simulink model "ApplicationSwComponentType11"  (R2024b)
settings: Solver=FixedStepDiscrete  StartTime=0.0  StopTime=10.0  FixedStep=0.01  RelTol=1e-3
model workspace (MAT data in the model file):
  ArTypedPerInstanceMemory = Simulink.Signal
  ArTypedPerInstanceMemory.Dimensions = 1
  ArTypedPerInstanceMemory.DimensionsMode = 'auto'
  ArTypedPerInstanceMemory.Complexity = 'real'
  ArTypedPerInstanceMemory.SampleTime = -1
  ArTypedPerInstanceMemory.SamplingMode = 'auto'
  ArTypedPerInstanceMemory.InitialValue = '-3'
  ArTypedPerInstanceMemory.DataType = 'int16'
  ConstantMemory = Simulink.Parameter
  ConstantMemory.Value = 3
  ConstantMemory.Complexity = 'real'
  ConstantMemory.Dimensions = [1 1]
  ConstantMemory.DataType = 'uint64'
  PerInstanceParameter = Simulink.Parameter
  PerInstanceParameter.Value = 5
  PerInstanceParameter.Complexity = 'real'
  PerInstanceParameter.Dimensions = [1 1]
  PerInstanceParameter.DataType = 'uint8'
  RPort_prm_Parameter = Simulink.Parameter
  RPort_prm_Parameter.Value = 0
  RPort_prm_Parameter.Complexity = 'real'
  RPort_prm_Parameter.Dimensions = [1 1]
  RPort_prm_Parameter.DataType = 'single'
  RPort_prm_Parameter1 = Simulink.Parameter
  RPort_prm_Parameter1.Value = 0
  RPort_prm_Parameter1.Complexity = 'real'
  RPort_prm_Parameter1.Dimensions = [1 1]
  RPort_prm_Parameter1.DataType = 'uint8'
  SharedParameter = Simulink.Parameter
  SharedParameter.Value = 5.5
  SharedParameter.Complexity = 'real'
  SharedParameter.Dimensions = [1 1]
  SharedParameter.DataType = 'single'
  StaticMemory = Simulink.Signal
  StaticMemory.Dimensions = 1
  StaticMemory.DimensionsMode = 'auto'
  StaticMemory.Complexity = 'real'
  StaticMemory.SampleTime = -1
  StaticMemory.SamplingMode = 'auto'
  StaticMemory.InitialValue = '9'
  StaticMemory.DataType = 'uint8'
settings Model: ParameterArgumentNames=PerInstanceParameter,RPort_prm_Parameter,RPort_prm_Parameter1  Creator=sss923875  LastModifiedBy=sss923875
settings DataIOCC: SaveFormat=StructureWithTime
settings OptimizationCC: DefaultParameterBehavior=Inlined  EnhancedBackFolding=on  PassReuseOutputArgsAs=Individual arguments  ZeroExternalMemoryAtStartup=off  ZeroInternalMemoryAtStartup=off  OptimizeBlockOrder=speed  DifferentSizesBufferReuse=on  OptimizationCustomize=off  EfficientTunableParamExpr=on
settings DebuggingCC: ParameterTunabilityLossMsg=error
settings HardwareCC: ProdLongLongMode=on
settings ModelReferenceCC: ModelReferenceNumInstancesAllowed=Single
settings SFSimCC: MATLABDynamicMemAlloc=off
settings RTWCC: Description=AUTOSAR  SystemTargetFile=autosar.tlc  GenCodeOnly=on  TemplateMakefile=ert_default_tmf  DataTypeReplacement=CDataTypesFixedWidth
settings CodeAppCC: ForceParamTrailComments=on  IgnoreCustomStorageClasses=off  OperatorAnnotations=on  SimulinkDataObjDesc=on  SFDataObjDesc=on  InsertBlockDesc=on
settings STFCustomTargetCC: TargetLangStandard=C99 (ISO)  MultiwordLength=256  ParMdlRefBuildCompliant=on  CompOptLevelCompliant=on  IncludeMdlTerminateFcn=off  CombineOutputUpdateFcns=on  SuppressErrorStatus=on  ERTCustomFileBanners=on  SupportNonFinite=off  SupportComplex=off  SupportContinuousTime=off  SupportNonInlinedSFcns=off  RemoveResetFunc=on  MATLABClassNameForMDSCustomization=Simulink.SoftwareTarget.ERTCustomization  AutosarCompliant=on  UseToolchainInfoCompliant=on  LookupTableObjectStructAxisOrder=2,1,3,4,...  LUTObjectStructOrderEvenSpacing=Size,Table,Breakpoints  SystemTargetFile=autosar.tlc
settings ERTTargetCC: TargetLangStandard=C99 (ISO)  ConcurrentExecutionCompliant=off  IncludeMdlTerminateFcn=off  SuppressErrorStatus=on  SupportNonFinite=off  SupportComplex=off  ModelStepFunctionPrototypeControlCompliant=off  CPPClassGenCompliant=off  AutosarCompliant=on  LookupTableObjectStructAxisOrder=2,1,3,4,...  LUTObjectStructOrderEvenSpacing=Size,Table,Breakpoints  ERTCustomFileTemplate=example_file_process.tlc  BooleanTrueId=TRUE  BooleanFalseId=FALSE

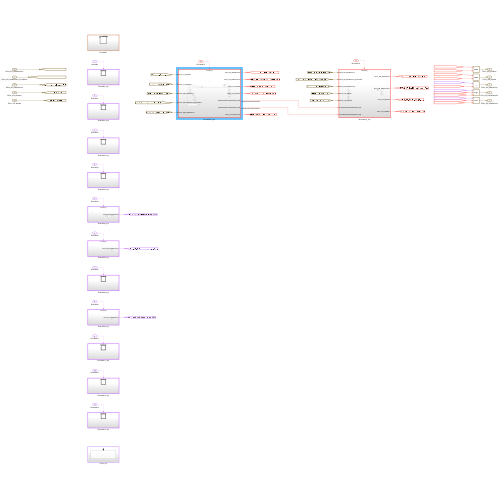
[thumbnail: Simulink's stored preview of the top-level diagram]
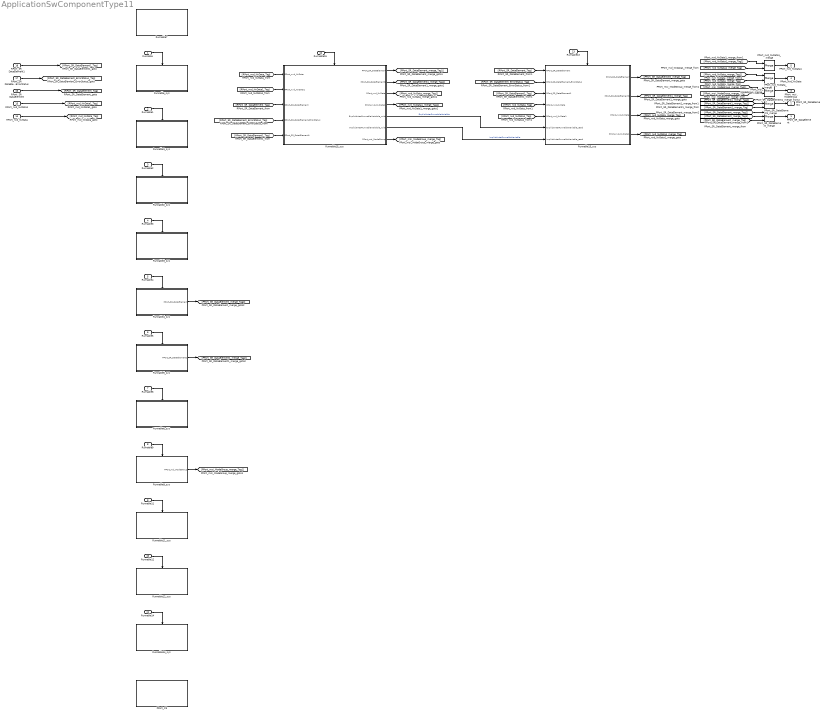
== system ApplicationSwComponentType11 ==
  Runnable : Inport  OutputFunctionCall=on
  Runnable1 : Inport  Port=2  OutputFunctionCall=on
  Runnable2 : Inport  Port=3  OutputFunctionCall=on
  Runnable3 : Inport  Port=4  OutputFunctionCall=on
  Runnable4 : Inport  Port=5  OutputFunctionCall=on
  Runnable5 : Inport  Port=6  OutputFunctionCall=on
  Runnable6 : Inport  Port=7  OutputFunctionCall=on
  Runnable9 : Inport  Port=8  OutputFunctionCall=on
  Runnable11 : Inport  Port=9  OutputFunctionCall=on
  Runnable12 : Inport  Port=10  OutputFunctionCall=on
  Runnable14 : Inport  Port=11  OutputFunctionCall=on
  Runnable15 : Inport  Port=12  SampleTime=0.01  OutputFunctionCall=on
  Runnable13 : Inport  Port=13  SampleTime=0.01  OutputFunctionCall=on
  RPort_nvd_NvData : Inport  Port=14  OutDataTypeStr=uint8  PortDimensions=1
  RPort_nvd_NvData1 : Inport  Port=15  OutDataTypeStr=double  PortDimensions=1
  RPort_SR_DataElement : Inport  Port=16  OutMin=0  OutMax=7  OutDataTypeStr=ApplicationPrimitiveDataType  PortDimensions=1
  RPort_SR_DataElement_ErrorStatus : Inport  Port=17  OutDataTypeStr=uint8  PortDimensions=1
  RPort_SR_DataElement1 : Inport  Port=18  OutDataTypeStr=uint32  PortDimensions=1
  PPort_CS : Subsystem
  PPort_SR_DataElement1_merge : Merge  Inputs=2+ 1
  PPort_SR_DataElement_merge : Merge  Inputs=2+ 1
  PPort_msi_ModeGroup_merge : Merge
  PPort_nvd_NvData1_merge : Merge
  PPort_nvd_NvData_merge : Merge
  Runnable11_sys : Subsystem
  Runnable12_sys : Subsystem
  Runnable13_sys : Subsystem
  Runnable14_sys : Subsystem
  Runnable15_sys : Subsystem
  Runnable1_sys : Subsystem
  Runnable2_sys : Subsystem
  Runnable3_sys : Subsystem
  Runnable4_sys : Subsystem
  Runnable5_sys : Subsystem
  Runnable6_sys : Subsystem
  Runnable7 : Subsystem
  Runnable9_sys : Subsystem
  Runnable_sys : Subsystem
  PPort_SR_DataElement : Outport  OutMin=0  OutMax=7  OutDataTypeStr=ApplicationPrimitiveDataType  PortDimensions=1
  PPort_SR_DataElement1 : Outport  Port=2  OutDataTypeStr=uint32  PortDimensions=1
  PPort_msi_ModeGroup : Outport  Port=3  OutDataTypeStr=Enum: ModeDeclarationGroup  PortDimensions=1
  PPort_nvd_NvData : Outport  Port=4  OutDataTypeStr=uint8  PortDimensions=1
  PPort_nvd_NvData1 : Outport  Port=5  OutDataTypeStr=double  PortDimensions=1
  wires:
  PPort_SR_DataElement_merge/1 -> PPort_SR_DataElement/1
  PPort_SR_DataElement1_merge/1 -> PPort_SR_DataElement1/1
  PPort_msi_ModeGroup_merge/1 -> PPort_msi_ModeGroup/1
  PPort_nvd_NvData_merge/1 -> PPort_nvd_NvData/1
  PPort_nvd_NvData1_merge/1 -> PPort_nvd_NvData1/1
  Runnable15_sys/5(ExplicitInterRunnableVariable_write) -> Runnable13_sys/6(ExplicitInterRunnableVariable_read)  "ExplicitInterRunnableVariable"
  Runnable15_sys/6(ImplicitInterRunnableVariable_write) -> Runnable13_sys/7(ImplicitInterRunnableVariable_read)  "ImplicitInterRunnableVariable"
  Runnable13_sys/4(PPort_nvd_NvData1) -> [PPort_nvd_NvData1_merge_Tag]
  [PPort_nvd_NvData1_merge_Tag] -> PPort_nvd_NvData1_merge/2
  Runnable15_sys/4(PPort_nvd_NvData1) -> [PPort_nvd_NvData1_merge_Tag1]
  [PPort_nvd_NvData1_merge_Tag1] -> PPort_nvd_NvData1_merge/1
  Runnable13_sys/3(PPort_nvd_NvData) -> [PPort_nvd_NvData_merge_Tag]
  [PPort_nvd_NvData_merge_Tag] -> PPort_nvd_NvData_merge/2
  Runnable15_sys/3(PPort_nvd_NvData) -> [PPort_nvd_NvData_merge_Tag1]
  [PPort_nvd_NvData_merge_Tag1] -> PPort_nvd_NvData_merge/1
  Runnable13_sys/2(PPort_SR_DataElement1) -> [PPort_SR_DataElement1_merge_Tag]
  [PPort_SR_DataElement1_merge_Tag] -> PPort_SR_DataElement1_merge/3
  Runnable13_sys/1(PPort_SR_DataElement) -> [PPort_SR_DataElement_merge_Tag]
  [PPort_SR_DataElement_merge_Tag] -> PPort_SR_DataElement_merge/3
  Runnable15_sys/7(PPort_msi_ModeGroup) -> [PPort_msi_ModeGroup_merge_Tag]
  [PPort_msi_ModeGroup_merge_Tag] -> PPort_msi_ModeGroup_merge/2
  Runnable9_sys/1(PPort_msi_ModeGroup) -> [PPort_msi_ModeGroup_merge_Tag1]
  [PPort_msi_ModeGroup_merge_Tag1] -> PPort_msi_ModeGroup_merge/1
  Runnable15_sys/2(PPort_SR_DataElement1) -> [PPort_SR_DataElement1_merge_Tag1]
  [PPort_SR_DataElement1_merge_Tag1] -> PPort_SR_DataElement1_merge/2
  Runnable5_sys/1(PPort_SR_DataElement1) -> [PPort_SR_DataElement1_merge_Tag2]
  [PPort_SR_DataElement1_merge_Tag2] -> PPort_SR_DataElement1_merge/1
  Runnable15_sys/1(PPort_SR_DataElement) -> [PPort_SR_DataElement_merge_Tag1]
  [PPort_SR_DataElement_merge_Tag1] -> PPort_SR_DataElement_merge/2
  Runnable4_sys/1(PPort_SR_DataElement) -> [PPort_SR_DataElement_merge_Tag2]
  [PPort_SR_DataElement_merge_Tag2] -> PPort_SR_DataElement_merge/1
  RPort_SR_DataElement1/1 -> [RPort_SR_DataElement1_Tag]
  [RPort_SR_DataElement1_Tag] -> Runnable15_sys/5(RPort_SR_DataElement1)
  [RPort_SR_DataElement1_Tag] -> Runnable13_sys/3(RPort_SR_DataElement1)
  RPort_SR_DataElement_ErrorStatus/1 -> [RPort_SR_DataElement_ErrorStatus_Tag]
  [RPort_SR_DataElement_ErrorStatus_Tag] -> Runnable15_sys/4(RPort_SR_DataElement_ErrorStatus)
  [RPort_SR_DataElement_ErrorStatus_Tag] -> Runnable13_sys/2(RPort_SR_DataElement_ErrorStatus)
  RPort_SR_DataElement/1 -> [RPort_SR_DataElement_Tag]
  [RPort_SR_DataElement_Tag] -> Runnable15_sys/3(RPort_SR_DataElement)
  [RPort_SR_DataElement_Tag] -> Runnable13_sys/1(RPort_SR_DataElement)
  RPort_nvd_NvData1/1 -> [RPort_nvd_NvData1_Tag]
  [RPort_nvd_NvData1_Tag] -> Runnable15_sys/2(RPort_nvd_NvData1)
  [RPort_nvd_NvData1_Tag] -> Runnable13_sys/5(RPort_nvd_NvData1)
  RPort_nvd_NvData/1 -> [RPort_nvd_NvData_Tag]
  [RPort_nvd_NvData_Tag] -> Runnable15_sys/1(RPort_nvd_NvData)
  [RPort_nvd_NvData_Tag] -> Runnable13_sys/4(RPort_nvd_NvData)
  Runnable/1 -> Runnable_sys/Trigger
  Runnable1/1 -> Runnable1_sys/Trigger
  Runnable2/1 -> Runnable2_sys/Trigger
  Runnable3/1 -> Runnable3_sys/Trigger
  Runnable4/1 -> Runnable4_sys/Trigger
  Runnable5/1 -> Runnable5_sys/Trigger
  Runnable6/1 -> Runnable6_sys/Trigger
  Runnable9/1 -> Runnable9_sys/Trigger
  Runnable11/1 -> Runnable11_sys/Trigger
  Runnable12/1 -> Runnable12_sys/Trigger
  Runnable14/1 -> Runnable14_sys/Trigger
  Runnable15/1 -> Runnable15_sys/Trigger
  Runnable13/1 -> Runnable13_sys/Trigger

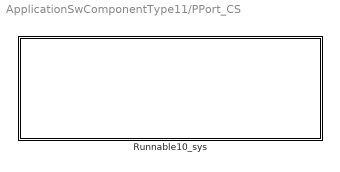
== system ApplicationSwComponentType11/PPort_CS ==
  Runnable10_sys : Subsystem

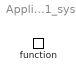
== system ApplicationSwComponentType11/Runnable11_sys ==
  function : TriggerPort  TriggerType=function-call  VariantControl=(inherit)

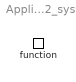
== system ApplicationSwComponentType11/Runnable12_sys ==
  function : TriggerPort  TriggerType=function-call  VariantControl=(inherit)

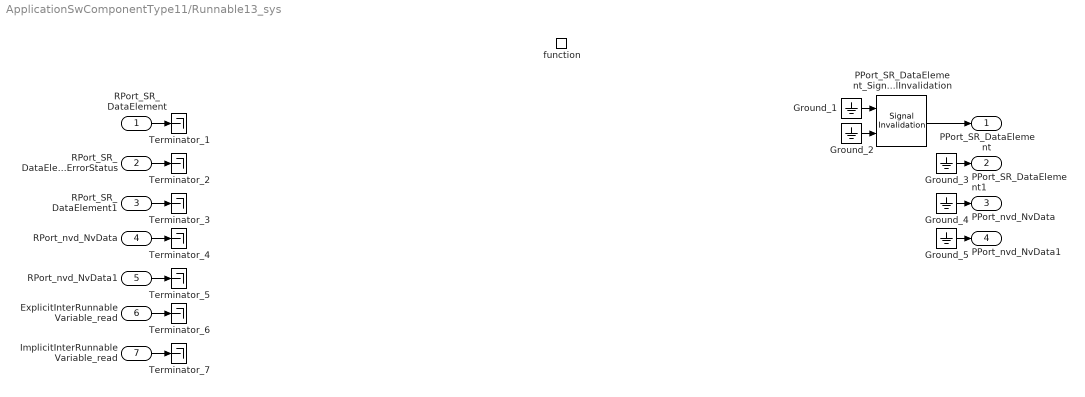
== system ApplicationSwComponentType11/Runnable13_sys ==
  RPort_SR_DataElement : Inport
  RPort_SR_DataElement_ErrorStatus : Inport  Port=2
  RPort_SR_DataElement1 : Inport  Port=3
  RPort_nvd_NvData : Inport  Port=4
  RPort_nvd_NvData1 : Inport  Port=5
  ExplicitInterRunnableVariable_read : Inport  Port=6
  ImplicitInterRunnableVariable_read : Inport  Port=7
  function : TriggerPort  TriggerType=function-call  VariantControl=(inherit)  SampleTimeType=periodic  SampleTime=-1
  Ground_{1..5} (5 alike) : Ground
  PPort_SR_DataElement_SignalInvalidation : SignalInvalidation
  Terminator_{1..7} (7 alike) : Terminator
  PPort_SR_DataElement : Outport
      settings: EnsureOutportIsVirtual=on
  PPort_SR_DataElement1 : Outport  Port=2
      settings: EnsureOutportIsVirtual=on
  PPort_nvd_NvData : Outport  Port=3
      settings: EnsureOutportIsVirtual=on
  PPort_nvd_NvData1 : Outport  Port=4
      settings: EnsureOutportIsVirtual=on
  wires:
  PPort_SR_DataElement_SignalInvalidation/1 -> PPort_SR_DataElement/1
  RPort_SR_DataElement/1 -> Terminator_1/1
  RPort_SR_DataElement_ErrorStatus/1 -> Terminator_2/1
  RPort_SR_DataElement1/1 -> Terminator_3/1
  RPort_nvd_NvData/1 -> Terminator_4/1
  RPort_nvd_NvData1/1 -> Terminator_5/1
  ExplicitInterRunnableVariable_read/1 -> Terminator_6/1
  ImplicitInterRunnableVariable_read/1 -> Terminator_7/1
  Ground_1/1 -> PPort_SR_DataElement_SignalInvalidation/1
  Ground_2/1 -> PPort_SR_DataElement_SignalInvalidation/2
  Ground_3/1 -> PPort_SR_DataElement1/1
  Ground_4/1 -> PPort_nvd_NvData/1
  Ground_5/1 -> PPort_nvd_NvData1/1

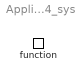
== system ApplicationSwComponentType11/Runnable14_sys ==
  function : TriggerPort  TriggerType=function-call  VariantControl=(inherit)

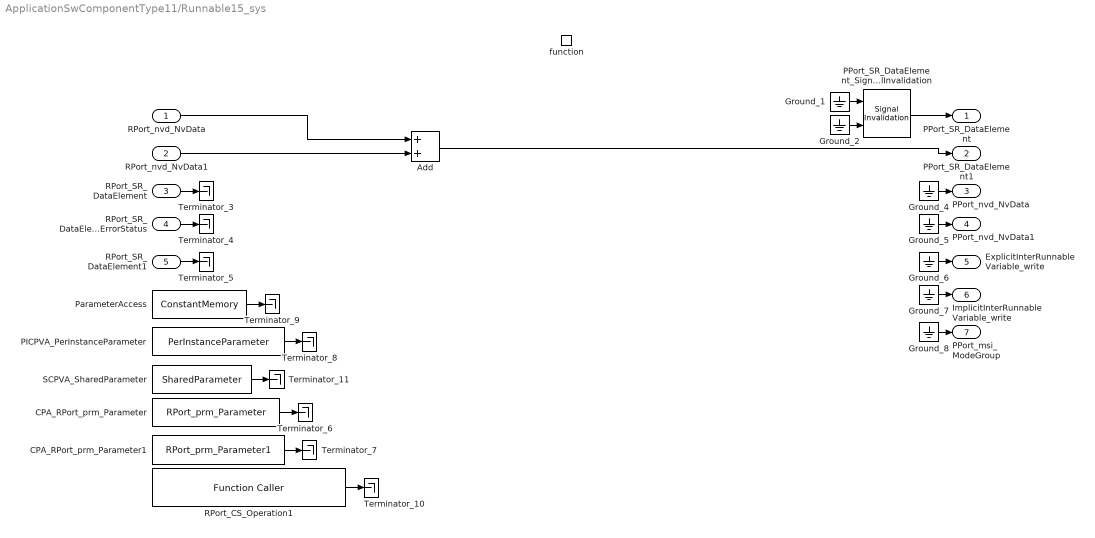
== system ApplicationSwComponentType11/Runnable15_sys ==
  RPort_nvd_NvData : Inport
  RPort_nvd_NvData1 : Inport  Port=2
  RPort_SR_DataElement : Inport  Port=3
  RPort_SR_DataElement_ErrorStatus : Inport  Port=4
  RPort_SR_DataElement1 : Inport  Port=5
  function : TriggerPort  TriggerType=function-call  VariantControl=(inherit)  SampleTimeType=periodic  SampleTime=-1
  Add : Sum
  CPA_RPort_prm_Parameter : Constant  Value=RPort_prm_Parameter
  CPA_RPort_prm_Parameter1 : Constant  Value=RPort_prm_Parameter1
  Ground_{1..2,4..8} (7 alike) : Ground
  PICPVA_PerInstanceParameter : Constant  Value=PerInstanceParameter
  PPort_SR_DataElement_SignalInvalidation : SignalInvalidation
  ParameterAccess : Constant  Value=ConstantMemory
  RPort_CS_Operation1 : FunctionCaller  FunctionPrototype=Argument = RPort_CS_Operation1()  OutputArgumentSpecifications=uint8(1)
  SCPVA_SharedParameter : Constant  Value=SharedParameter
  Terminator_{3..11} (9 alike) : Terminator
  PPort_SR_DataElement : Outport
      settings: EnsureOutportIsVirtual=on
  PPort_SR_DataElement1 : Outport  Port=2
      settings: EnsureOutportIsVirtual=on
  PPort_nvd_NvData : Outport  Port=3
      settings: EnsureOutportIsVirtual=on
  PPort_nvd_NvData1 : Outport  Port=4
      settings: EnsureOutportIsVirtual=on
  ExplicitInterRunnableVariable_write : Outport  Port=5  OutDataTypeStr=boolean  PortDimensions=1
  ImplicitInterRunnableVariable_write : Outport  Port=6  OutDataTypeStr=int16  PortDimensions=1
  PPort_msi_ModeGroup : Outport  Port=7
      settings: EnsureOutportIsVirtual=on
  wires:
  PPort_SR_DataElement_SignalInvalidation/1 -> PPort_SR_DataElement/1
  RPort_nvd_NvData/1 -> Add/1
  RPort_nvd_NvData1/1 -> Add/2
  RPort_SR_DataElement/1 -> Terminator_3/1
  RPort_SR_DataElement_ErrorStatus/1 -> Terminator_4/1
  RPort_SR_DataElement1/1 -> Terminator_5/1
  CPA_RPort_prm_Parameter/1 -> Terminator_6/1
  CPA_RPort_prm_Parameter1/1 -> Terminator_7/1
  PICPVA_PerInstanceParameter/1 -> Terminator_8/1
  Ground_1/1 -> PPort_SR_DataElement_SignalInvalidation/1
  Ground_2/1 -> PPort_SR_DataElement_SignalInvalidation/2
  ParameterAccess/1 -> Terminator_9/1
  RPort_CS_Operation1/1 -> Terminator_10/1
  SCPVA_SharedParameter/1 -> Terminator_11/1
  Add/1 -> PPort_SR_DataElement1/1
  Ground_4/1 -> PPort_nvd_NvData/1
  Ground_5/1 -> PPort_nvd_NvData1/1
  Ground_6/1 -> ExplicitInterRunnableVariable_write/1
  Ground_7/1 -> ImplicitInterRunnableVariable_write/1
  Ground_8/1 -> PPort_msi_ModeGroup/1

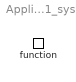
== system ApplicationSwComponentType11/Runnable1_sys ==
  function : TriggerPort  TriggerType=function-call  VariantControl=(inherit)

== system ApplicationSwComponentType11/Runnable2_sys ==
  function : TriggerPort  TriggerType=function-call  VariantControl=(inherit)

== system ApplicationSwComponentType11/Runnable3_sys ==
  function : TriggerPort  TriggerType=function-call  VariantControl=(inherit)

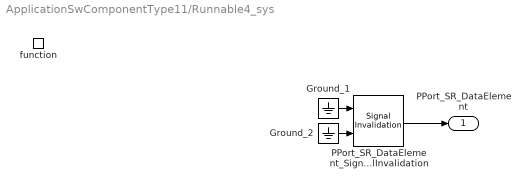
== system ApplicationSwComponentType11/Runnable4_sys ==
  function : TriggerPort  TriggerType=function-call  VariantControl=(inherit)
  Ground_1 : Ground
  Ground_2 : Ground
  PPort_SR_DataElement_SignalInvalidation : SignalInvalidation
  PPort_SR_DataElement : Outport
      settings: EnsureOutportIsVirtual=on
  wires:
  PPort_SR_DataElement_SignalInvalidation/1 -> PPort_SR_DataElement/1
  Ground_1/1 -> PPort_SR_DataElement_SignalInvalidation/1
  Ground_2/1 -> PPort_SR_DataElement_SignalInvalidation/2

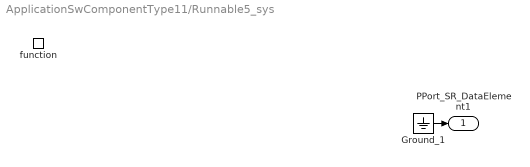
== system ApplicationSwComponentType11/Runnable5_sys ==
  function : TriggerPort  TriggerType=function-call  VariantControl=(inherit)
  Ground_1 : Ground
  PPort_SR_DataElement1 : Outport
      settings: EnsureOutportIsVirtual=on
  wires:
  Ground_1/1 -> PPort_SR_DataElement1/1

== system ApplicationSwComponentType11/Runnable6_sys ==
  function : TriggerPort  TriggerType=function-call  VariantControl=(inherit)

== system ApplicationSwComponentType11/Runnable7 ==
  Event Listener : EventListener  EventName=reset

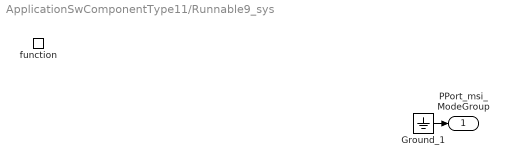
== system ApplicationSwComponentType11/Runnable9_sys ==
  function : TriggerPort  TriggerType=function-call  VariantControl=(inherit)
  Ground_1 : Ground
  PPort_msi_ModeGroup : Outport
      settings: EnsureOutportIsVirtual=on
  wires:
  Ground_1/1 -> PPort_msi_ModeGroup/1

== system ApplicationSwComponentType11/Runnable_sys ==
  function : TriggerPort  TriggerType=function-call  VariantControl=(inherit)

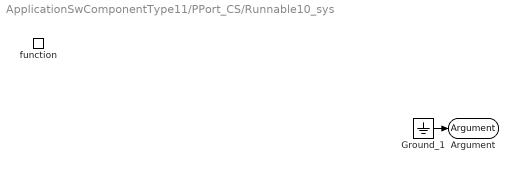
== system ApplicationSwComponentType11/PPort_CS/Runnable10_sys ==
  function : TriggerPort  TriggerType=function-call  IsSimulinkFunction=on  FunctionName=ApplicationSwComponentType_Runnable10  VariantControl=(inherit)
  Ground_1 : Ground
  Argument : ArgOut  OutDataTypeStr=uint8  ArgumentName=Argument
  wires:
  Ground_1/1 -> Argument/1
